simulink model "base"  (R2018b)
settings: Solver=VariableStepAuto  StartTime=0.0  StopTime=10.0  RelTol=1e-3
libraries: cstblocks x1
settings Model: Creator=Abraham Pérez  LastModifiedBy=Abraham Pérez

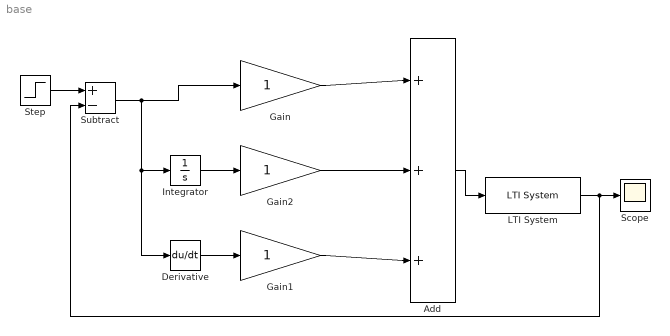
== system base ==
  Add : Sum  Inputs=+++
  Derivative : Derivative
  Gain : Gain
  Gain1 : Gain
  Gain2 : Gain
  Integrator : Integrator
  LTI System : cstblocks/LTI System  sys=tf(1,[1 1])  IC=[]
  Scope : Scope
  Step : Step  SampleTime=0
  Subtract : Sum  Inputs=+-
  wires:
  Add/1 -> LTI System/1
  LTI System/1 -> Subtract/2, Scope/1
  Gain1/1 -> Add/3
  Gain2/1 -> Add/2
  Gain/1 -> Add/1
  Integrator/1 -> Gain2/1
  Step/1 -> Subtract/1
  Subtract/1 -> Derivative/1, Integrator/1, Gain/1
  Derivative/1 -> Gain1/1
